simulink model "radia_rlc_resonance_plant"  (R2026a)
settings: Solver=ode45  StopTime=0.02  MaxStep=2e-5  RelTol=1e-9  AbsTol=1e-11
PreLoadFcn:
  | R_ohm=2; L_H=10e-3; C_F=2.5e-6;
settings Model: Creator=Administrator  LastModifiedBy=Administrator

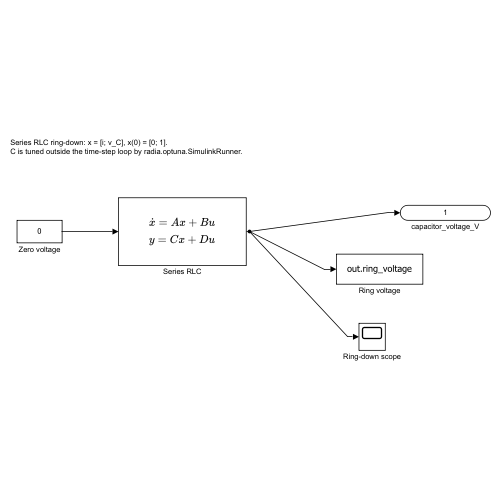
[thumbnail: Simulink's stored preview of the top-level diagram]
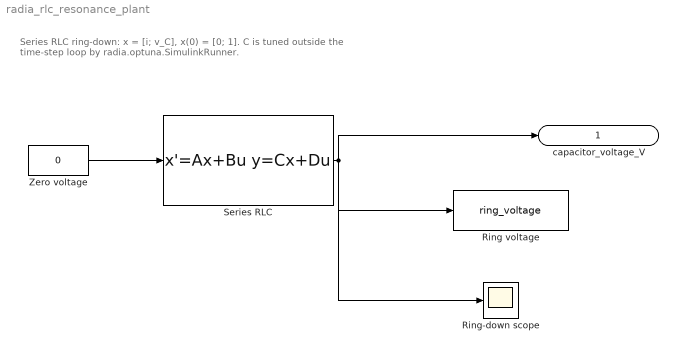
== system radia_rlc_resonance_plant ==
  note: Series RLC ring-down: x = [i; v_C], x(0) = [0; 1].
      | C is tuned outside the time-step loop by radia.optuna.SimulinkRunner.
  Ring voltage : ToWorkspace  VariableName=ring_voltage  SaveFormat=Timeseries  SampleTime=-1
  Ring-down scope : Scope
  Series RLC : StateSpace  A=[-R_ohm/L_H -1/L_H; 1/C_F 0]  B=[1/L_H; 0]  C=[0 1]  D=0  InitialCondition=[0; 1]
  Zero voltage : Constant  Value=0
  capacitor_voltage_V : Outport
  wires:
  Zero voltage/1 -> Series RLC/1
  Series RLC/1 -> capacitor_voltage_V/1, Ring voltage/1, Ring-down scope/1
